simulink model "part2"  (R2025a)
settings: Solver=ode4  StartTime=0.0  StopTime=500  FixedStep=0.1  RelTol=1e-3
values from neighbouring files (symbols this model uses):
  A_f = diag([1/t1 1/t2 1/t3])    [reference_model.m]
  A_w = [zeros(3,3), eye(3); -omega_ekf^2, -2*lambda_ekf*omega_ekf]    [kalman.m]
  Aw = [zeros(3,3), eye(3); -omega*omega, -2*lambda*omega]    [observer.m]
  B_ekf = [zeros(6,3);zeros(3,3); zeros(3,3);M_inv]    [kalman.m]
  Cw = [zeros(3,3), eye(3)]    [observer.m]
  D_diag = D    [observer.m]
  E_ekf = [E_w zeros(6,3) ... (first row only)    [kalman.m]
  G = zeros(3,3)    [kalman.m]
  Gamma = diag([w1^2, w2^2, w3^2])    [reference_model.m]
  H_ekf = [C_w eye(3) zeros(3,3) zeros(3,3)]    [kalman.m]
  h_ekf = 0.1    [kalman.m]
  K1 = [diag([k1, k2, k3]); diag([k4, k5, k6])]    [observer.m]
  K2 = diag([k7, k8, k9])    [observer.m]
  K3 = 0.1* K4    [observer.m]
  K4 = diag([M_diag(1,1), M_diag(1,1), M_diag(1,1)])*1e-1    [observer.m]
  K_w_ekf = diag(Kwi)    [kalman.m]
  Kd = diag([Kd_t(1,1), Kd_t(2,2), Kd_t(3,3)])    [PID.m]
  Ki = diag([Ki_t(1,1), Ki_t(2,2), Ki_t(3,3)])    [PID.m]
  Kp = diag([Kp_t(1,1), Kp_t(2,2), Kp_t(3,3)])    [PID.m]
  lambda_ekf = diag(zeta)    [kalman.m]
  M_diag = [Mtot(1,1), 0, 0 ... (first row only)    [observer.m]
  M_inv = inv(M_3)    [kalman.m]    (also in observer.m = inv(M_diag))
  mu = 0.001    [init.m]
  mu_direction = 0.03    [init.m]
  Omega = diag([2*zeta1*w1, 2*zeta2*w2, 2*zeta3*w3])    [reference_model.m]
  omega_ekf = diag([w, w, w])    [kalman.m]
  P_0 = eye(15)    [kalman.m]
  Q_ekf = diag([0.001, 0.001, 0.001, 1e8, 1e8, 1e9])    [kalman.m]
  R_ekf = diag([1, 5, 0.01])    [kalman.m]
  rate = [rate(1), rate(2), rate(2), rate(3), rate(4),rate(4), rate(5), rate(5)]    [thrust_allocation.m]
  rotationspeed = [0 rotationspeed(1) 0 rotationspeed(2) rotationspeed(3)]    [thrust_allocation.m]
  step1 = 50    [reference_model.m]
  step2 = 1.4    [reference_model.m]
  step3 = 1.2    [reference_model.m]
  T_b_ekf = 1000*diag([1, 1, 1])    [kalman.m]
  Tb_inv = inv(Tb)    [observer.m]
  thrust = [thrust(1), thrust(2), thrust(2), thrust(3), thrust(4), thrust(4), thrust(5), thrust(5)]    [thrust_allocation.m]
  U_10 = 10    [init.m]
  U_angle = 180    [init.m]
  U_mean = U_10*(5/2)*sqrt(K)*log(z/z0)    [init.m]
  W = diag([10, 1, 1, 10, 1, 1, 1, 1])    [thrust_allocation.m]
  w = 0.005    [init.m]    (also in kalman.m = 0.698131700798)
  x_0 = zeros(1,15)    [kalman.m]
  xpos = [thrusters.xposition]    [thrust_allocation.m]
  ypos = [thrusters.yposition]    [thrust_allocation.m]
undefined symbols (not defined in the file or in its folder): alpha, C_pitch, C_roll, C_yaw, Cx, Cy, Cz, Hoerner, thrusters, vessel, wind_coeff
libraries: marine_gnc x9, simulink x8, dspsigops x3, marine_hydro x2, simulink_extras x2
(part 2 of 2)

== matlab function part2/Observer/Extended kalmanfilter/Kalman predictor ==
  data: x_predict output; P_predict output; tau input; x_hat input; P_hat input; M_diag input; D_diag input; A_w parameter; B_ekf parameter; E_ekf parameter; Q_ekf parameter; R_ekf parameter; h_ekf parameter; omega_ekf parameter; lambda_ekf parameter; K_w_ekf parameter; G1 input; T_b_ekf parameter
function [x_predict, P_predict] = fcn(tau, x_hat, P_hat, M_diag, D_diag, A_w, B_ekf, E_ekf, Q_ekf, R_ekf, h_ekf, omega_ekf, lambda_ekf, K_w_ekf, G1, T_b_ekf)
%where x_est and P_est is the state observer
%%Definition for Extended Kalman filter
D_3= D_diag;
M_3= M_diag;
M_inv=inv(M_3());
%jacobi(x_hat, A_w, inv(T_b_ekf), M_inv, D_3);
%%Jacobi calculated by Matlab
%x1=x_hat1
function[J] = jacobi(x_hat, A_w1, inv_Tb, M_inv1, D_31)
J =[A_w1(1,1),    0,    0,    0,    0,    0,                  0,                  0,                                                                                     0,               0,              0,       0,            0,            0,            0;
   0, A_w1(2,2),    0,    0,    0,    0,                  0,                  0,                                                                                     0,               0,              0,       0,            0,            0,            0;
   0,    0, A_w1(3,3),    0,    0,    0,                  0,                  0,                                                                                     0,               0,              0,       0,            0,            0,            0;
   0,    0,    0, A_w1(4,4),    0,    0,                  0,                  0,                                                                                     0,               0,              0,       0,            0,            0,            0;
   0,    0,    0,    0, A_w1(5,5),    0,                  0,                  0,                                                                                     0,               0,              0,       0,            0,            0,            0;
   0,    0,    0,    0,    0, A_w1(6,6),                  0,                  0,                                                                                     0,               0,              0,       0,            0,            0,            0;
   0,    0,    0,    0,    0,    0,                  0,                  0,                                                           - x_hat(14)*cos(x_hat(9)) - x_hat(13)*sin(x_hat(9)),               0,              0,       0,      cos(x_hat(9)),     -sin(x_hat(9)),            0;
   0,    0,    0,    0,    0,    0,                  0,                  0,                                                             x_hat(13)*cos(x_hat(9)) - x_hat(14)*sin(x_hat(9)),               0,              0,       0,      sin(x_hat(9)),      cos(x_hat(9)),            0;
   0,    0,    0,    0,    0,    0,                  0,                  0,                                                                                     0,               0,              0,       0,            0,            0,            1;
   0,    0,    0,    0,    0,    0,                  0,                  0,                                                                                     0,         -inv_Tb(1,1),              0,       0,            0,            0,            0;
   0,    0,    0,    0,    0,    0,                  0,                  0,                                                                                     0,               0,        -inv_Tb(2,2),       0,            0,            0,            0;
   0,    0,    0,    0,    0,    0,                  0,                  0,                                                                                     0,               0,              0, -inv_Tb(3,3),            0,            0,            0;
   0,    0,    0,    0,    0,    0, -G1(1,1)*M_inv1(1,1)*cos(x_hat(9)), -G1(1,1)*M_inv1(1,1)*sin(x_hat(9)), M_inv1(1,1)*x_hat(11)*cos(x_hat(9)) - M_inv1(1,1)*x_hat(10)*sin(x_hat(9)) - G1(1,1)*M_inv1(1,1)*x_hat(8)*cos(x_hat(9)) + G1(1,1)*M_inv1(1,1)*x_hat(7)*sin(x_hat(9)),  M_inv1(1,1)*cos(x_hat(9)), M_inv1(1,1)*sin(x_hat(9)),       0, -D_31(1,1)*M_inv1(1,1),            0,            0;
   0,    0,    0,    0,    0,    0,  G1(2,2)*M_inv1(2,2)*sin(x_hat(9)), -G1(2,2)*M_inv1(2,2)*cos(x_hat(9)), G1(2,2)*M_inv1(2,2)*x_hat(7)*cos(x_hat(9)) - M_inv1(2,2)*x_hat(11)*sin(x_hat(9)) - M_inv1(2,2)*x_hat(10)*cos(x_hat(9)) + G1(2,2)*M_inv1(2,2)*x_hat(8)*sin(x_hat(9)), -M_inv1(2,2)*sin(x_hat(9)), M_inv1(2,2)*cos(x_hat(9)),       0,            0, -D_31(2,2)*M_inv1(2,2),            0;
   0,    0,    0,    0,    0,    0,                  0,                  0,                                                                            -G1(3,3)*M_inv1(3,3),               0,              0,  M_inv1(3,3),            0,            0, -D_31(3,3)*M_inv1(3,3)];
end


phi = eye(15)+ h_ekf*jacobi(x_hat, A_w, inv(T_b_ekf), M_inv, D_3);
gamma=h_ekf*E_ekf;
P_predict=phi*P_hat*phi'+ gamma*Q_ekf*gamma';
x_predict=x_hat+h_ekf*(f(x_hat, A_w, T_b_ekf, M_inv, D_3)+B_ekf*tau);


function f = f(x_hat, A_w, T_b_ekf, M_inv, D_3)
    Tb_inv = inv(T_b_ekf);

    f = zeros(15,1);
    f(1:6,1) = A_w*x_hat(1:6,1);
    f(7:9,1) = R(x_hat(9,1))*x_hat(13:15,1);
    f(10:12,1) = -(Tb_inv)*x_hat(10:12,1);
    f(13:15,1) = (-M_inv*D_3*x_hat(13:15,1)) + M_inv*(R(x_hat(9,1)))'*x_hat(10:12,1);
end

function Rotation = R(psi)
     Rotation = [cos(psi) -sin(psi) 0;
            sin(psi) cos(psi) 0;
            0   0   1];
end

end
